simulink model "Controller_Simulation"  (R2022b)
settings: Solver=ode4  StartTime=0.0  StopTime=40  FixedStep=0.01  RelTol=1e-3
settings Model: PacingRate=0.100000  Creator=Sahil Gaurkar  LastModifiedBy=Sahil Gaurkar

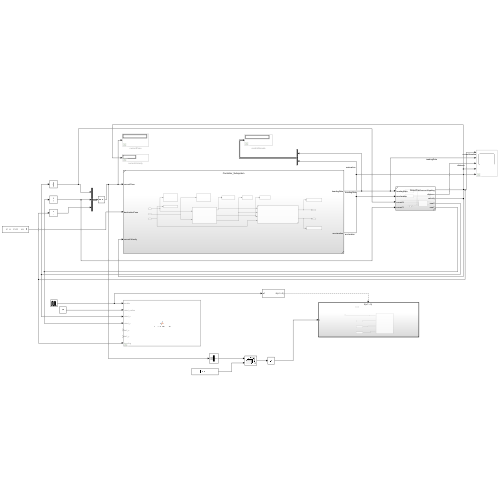
[thumbnail: Simulink's stored preview of the top-level diagram]
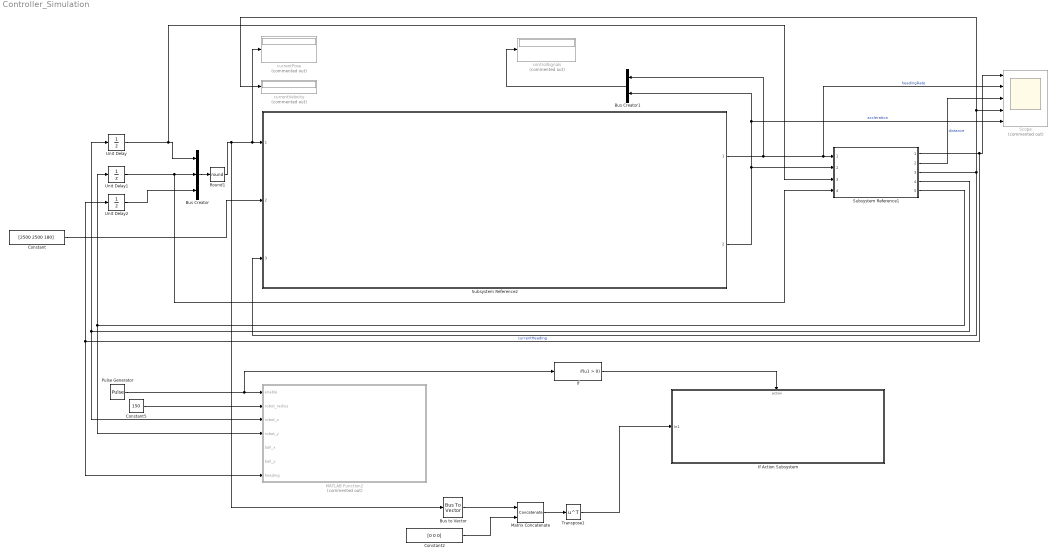
== system Controller_Simulation ==
  Bus Creator : BusCreator  Inputs=3
  Bus Creator1 : BusCreator  Inputs=2
  Bus to Vector : BusToVector
  Constant : Constant  Value=[2500 2500 180]
  Constant2 : Constant  Value=[0 0 0]
  Constant5 : Constant  Value=150
  If : If  ShowElse=off
  If Action Subsystem : Subsystem  TreatAsAtomicUnit=on
  MATLAB Function2 : MATLAB Function  Commented=on  InitFcn=|  TreatAsAtomicUnit=on
      | figure(1); 
      | clf;
      | hold on; 
      | grid on; 
      | axis([-45,45,-30,30]);
  Matrix Concatenate : Concatenate  Mode=Multidimensional array  ConcatenateDimension=2
  Pulse Generator : DiscretePulseGenerator  PulseType=Time based  Period=1
  Round1 : Rounding  Operator=round
  Scope : Scope  Commented=on  NumInputPorts=5
  Subsystem Reference1 : Subsystem  ReferencedSubsystem=RobotPlant
  Subsystem Reference2 : Subsystem  ReferencedSubsystem=Controller_Subsystem
  Transpose1 : Math  Operator=transpose
  Unit Delay : UnitDelay  InitialCondition=1000  SampleTime=-1  HasFrameUpgradeWarning=on
  Unit Delay1 : UnitDelay  InitialCondition=1000  SampleTime=-1  HasFrameUpgradeWarning=on
  Unit Delay2 : UnitDelay  InitialCondition=-20  SampleTime=-1  HasFrameUpgradeWarning=on
  controlSignals : Display  Commented=on
  currentPose : Display  Commented=on
  currentVelocity : Display  Commented=on
  wires:
  Unit Delay2/1 -> Bus Creator/3
  Constant/1 -> Subsystem Reference2/2
  Unit Delay1/1 -> Subsystem Reference1/4, Bus Creator/2
  Subsystem Reference2/2 -> Bus Creator1/2, Scope/5, Subsystem Reference1/2  "accleration"
  Bus Creator1/1 -> controlSignals/1
  Bus Creator/1 -> Round1/1
  Subsystem Reference2/1 -> Scope/2, Subsystem Reference1/1, Bus Creator1/1  "headingRate"
  Subsystem Reference1/1 -> Scope/1, MATLAB Function2/7(heading), Unit Delay2/1  "currentHeading"
  Subsystem Reference1/2 -> Scope/3  "distance"
  Subsystem Reference1/3 -> Subsystem Reference2/3, Scope/4, currentVelocity/1
  Subsystem Reference1/5 -> Unit Delay1/1, MATLAB Function2/4(robot_y)
  Constant5/1 -> MATLAB Function2/2(robot_radius)
  Subsystem Reference1/4 -> Unit Delay/1, MATLAB Function2/3(robot_x)
  Unit Delay/1 -> Bus Creator/1, Subsystem Reference1/3
  Round1/1 -> Subsystem Reference2/1, currentPose/1, Bus to Vector/1
  Pulse Generator/1 -> If/1, MATLAB Function2/1(enable)
  If/1 -> If Action Subsystem/Action
  Bus to Vector/1 -> Matrix Concatenate/1
  Constant2/1 -> Matrix Concatenate/2
  Matrix Concatenate/1 -> Transpose1/1
  Transpose1/1 -> If Action Subsystem/1(In1)

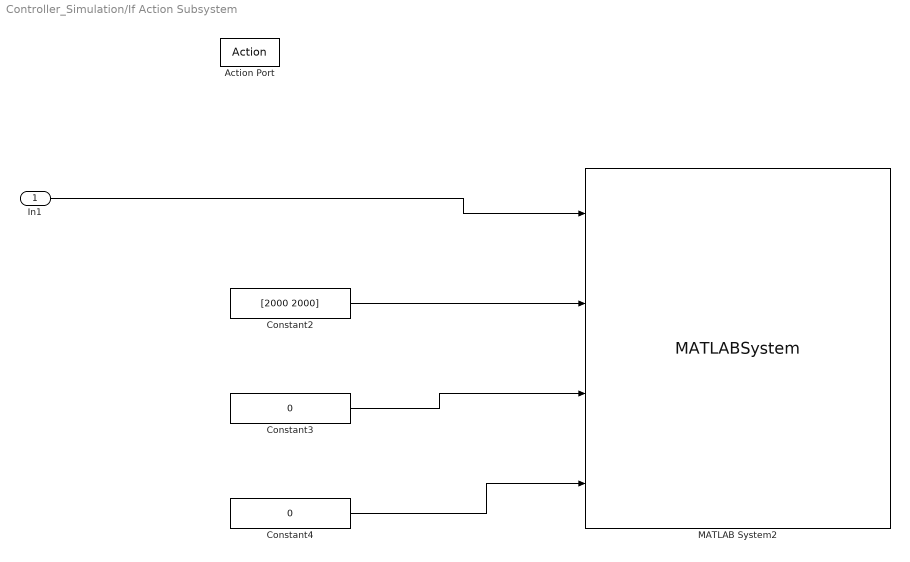
== system Controller_Simulation/If Action Subsystem ==
  In1 : Inport
  Action Port : ActionPort  ActionPortLabel=if(u1 > 0)
  Constant2 : Constant  Value=[2000 2000]
  Constant3 : Constant  Value=0
  Constant4 : Constant  Value=0
  MATLAB System2 : MATLABSystem  System=simulation_window_3  pitch_length=9000  pitch_width=6000  centre_circle_diameter=1500  border_strip_width=1000  goal_area_length=1000  goal_area_width=1000  penalty_area_length=1000  penalty_area_width=3000  goal_width=1000  goal_depth=500  SimulateUsing=Code generation
      mask Type: simulation_window_3
      mask Display:
      | disp('simulation_window_3');
      | port_label('input',1,'robot_coordinates');
      | port_label('input',2,'ball_coordinates');
      | port_label('input',3,'scoreTeam1');
      | port_label('input',4,'scoreTeam2');
  wires:
  Constant4/1 -> MATLAB System2/4
  Constant3/1 -> MATLAB System2/3
  Constant2/1 -> MATLAB System2/2
  In1/1 -> MATLAB System2/1

== matlab function Controller_Simulation/MATLAB Function2 ==
  data: enable input; robot_radius input; robot_x input; robot_y input; ball_x input; ball_y input; heading input
function plotRobotAndBall(enable, robot_radius, robot_x, robot_y, ball_x, ball_y, heading)

if enable == 1
    figure(1);
    clf;
    hold on;
    grid on;
    axis([-9000,9000,-9000,9000]);

    theta = linspace(0, 2*pi, 360);
    heading_line_length = 300; % L

    % equation of circle for representing robot
    robot_rep_x = robot_radius * cos(theta);
    robot_rep_y = robot_radius * sin(theta);

    heading_line_x = cos((heading*pi)/180) * heading_line_length;
    heading_line_y = sin((heading*pi)/180) * heading_line_length;

    % Draw circle around current location of robot
    plot((robot_rep_x + robot_x), (robot_rep_y + robot_y), 'Color', 'b');

    % Draw line from center of robot in the direction of the current heading
    line([robot_x,  robot_x + heading_line_x], [robot_y, robot_y + heading_line_y], 'color', 'b');

    % Plot ball
    plot(ball_x, ball_y,'Color','r','Marker','o')

    drawnow();

end


end
